simulink model "detector10"  (Simulink 2.20)
settings: Solver=ode45  StartTime=0.0  StopTime=10.0  RelTol=1e-3  AbsTol=1e-6
undefined symbols (not defined in the file): firls
libraries: BufferedDSP x6, dspbuff x1, WinAudio x1
settings Model: ConsistencyChecking=off  RTWPlaceOutputsASAP=off  RTWTemplateMakefile=c:\nfc\matlab\simulink\grt_vc_sgm.tmf  RTWMakeCommand="make_rtw USER_SRCS=\"winmm.lib\" USER_INCLUDES=\"-Ic:\\nfc\\matlab\\Simulink\\BufferedDSP\\src\\rtw\""

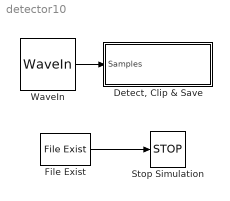
== system detector10 ==
  "Detect, Clip & Save" : Subsystem  mask(DetectClipNSave){buffersize=8192, f0=2500, f1=5000, threshold=1.8, numChannels=1, col_major=0, fs=22050}
      mask prompts: buffersize "Buffer Size:"; f0 "Lower Frequency (Hz):"; f1 "Upper Frequency (Hz):"; numChannels "Number of Channels:"; col_major "Column major channel order:"; fs "Sample Rate (Hz):"
      mask help: Detects acoustic events in a frequency band, clips, and saves them to disk.
      mask Help: Detects acoustic events in a frequency band, clips, and saves them to disk.
  File Exist : BufferedDSP/Other/File Exist  filename=c:\stop.txt  sampleTime=3*8192/22050
  Stop Simulation : Stop
  WaveIn : WinAudio/WaveIn  sampleRateLit=22050  sampleWidthLit=16  stereo=off  col_major=0  buffersize=8192  bufTime=12
  wires:
  WaveIn/1 -> "Detect, Clip & Save"/1(Samples)
  File Exist/1 -> Stop Simulation/1

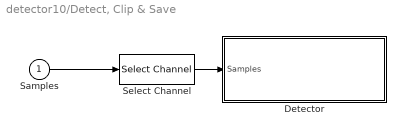
== system detector10/Detect, Clip & Save ==
  Samples : Inport  Port=1  PortWidth=buffersize * numChannels  SampleTime=-1
  Detector : Subsystem  mask(Detector){buffersize=buffersize, f0=f0, f1=f1, filterLength=100, threshold=threshold, numChannels=1, col_major=col_major, fs=fs}
      mask prompts: buffersize "Buffer Size:"; f0 "Lower Frequency (Hz):"; f1 "Upper Frequency (Hz):"; filterLength "Filter Length:"; numChannels "Number of Channels:"; col_major "Column major channel order:"; fs "Sample Rate:"
      mask help: Examines band-limited energy for events.
  Select Channel : BufferedDSP/Multichannel/Select Channel  buffersize=buffersize  selectChannel=1  numChannels=numChannels  col_major=col_major
  wires:
  Select Channel/1 -> Detector/1(Samples)
  Samples/1 -> Select Channel/1

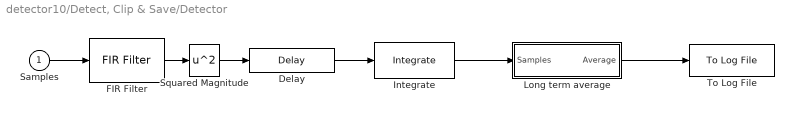
== system detector10/Detect, Clip & Save/Detector ==
  Samples : Inport  Port=1  PortWidth=buffersize *numChannels  SampleTime=-1
  Delay : BufferedDSP/Memory/Delay  buffersize=buffersize  delay=7179+0.06*fs  numChannels=1  col_major=1
  FIR Filter : BufferedDSP/Filter/Row Major/FIR Filter  input_width=buffersize  nfft_in=2*buffersize  h=firls(filterLength-1,[0 f0-100 f0 f1 f1+100 fs/2]/(fs/2),[0,0,1,1,0,0])  numChannels=numChannels
  Integrate : BufferedDSP/Filter/Integrate  buffersize=buffersize  integration_time=round(.050*fs)  normalize=on  initial_value=0  numChannels=numChannels  col_major=col_major
  Long term average : Subsystem
  Squared Magnitude : Math  Operator=square
  To Log File : BufferedDSP/Other/To Log File  sample_time=60  input_width=1  time_stamp_option=Local time  filename=c:\Logfile.txt
  wires:
  FIR Filter/1 -> Squared Magnitude/1
  Samples/1 -> FIR Filter/1
  Long term average/1(Average) -> To Log File/1
  Delay/1 -> Integrate/1
  Integrate/1 -> Long term average/1(Samples)
  Squared Magnitude/1 -> Delay/1

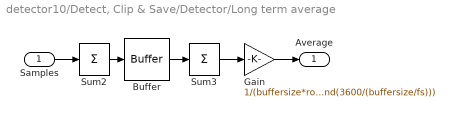
== system detector10/Detect, Clip & Save/Detector/Long term average ==
  Samples : Inport  Port=1  PortWidth=-1  SampleTime=-1
  Buffer : dspbuff/Buffer  N=round(3600/(buffersize/fs))  V=0  Ts=buffersize/fs  ic=0
  Gain : Gain  Gain=1/(buffersize*round(3600/(buffersize/fs)))
  Sum2 : Sum  Inputs=1
  Sum3 : Sum  Inputs=1
  Average : Outport  Port=1
  wires:
  Sum2/1 -> Buffer/1
  Buffer/1 -> Sum3/1
  Sum3/1 -> Gain/1
  Gain/1 -> Average/1
  Samples/1 -> Sum2/1
